simulink model "chienSearch_test"  (R2021a)
settings: Solver=VariableStepAuto  StartTime=0.0  StopTime=10.0  RelTol=1e-3
settings Model: Creator=Jackie Smedley  LastModifiedBy=Jackie Smedley

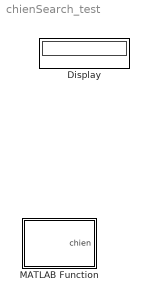
== system chienSearch_test ==
  Display : Display
  MATLAB Function : MATLAB Function  TreatAsAtomicUnit=on
  wires:
  ? -> Display/1

== matlab function chienSearch_test/MATLAB Function ==
  data: chien output
function chien = fcn()
primPoly = [1, 0, 1, 1];
m = 3;
lambda = [-1 -1 -1 -1 -1 5 2 0];
degree = 2;
gf = GenerateGF2m(primPoly, m);
chien = chienSearch(lambda, degree, gf);
end
